simulink model "FOC_AM263X"  (R2024b)
settings: Solver=FixedStepAuto  StartTime=0.0  StopTime=10.0  RelTol=1e-3
model workspace: external: MATLAB File C:\Users\A0499511\Documents\MATLAB\Examples\R2024b\c2b\SensorlessfocUsingC2000ProcessorsExample\FOC_AM263X_Data.m (data not in the file)
values from neighbouring files (symbols this model uses):
  acceleration = 20000/PU_System.N_base    [FOC_AM263PX_Datascript.m]    (also in FOC_AM263X_Datascript.m)
  inverter = mcb_SetInverterParameters('BoostXL-DRV8305')    [FOC_AM263PX_Datascript.m]    (also in FOC_AM263X_Datascript.m)
  PI_params = mcb.internal.SetControllerParameters(pmsm,inverter,PU_System,T_pwm,2*Ts,Ts_speed)    [FOC_AM263PX_Datascript.m]    (also in FOC_AM263X_Datascript.m)
  pmsm = mcb_SetPMSMMotorParameters('BLY171D')    [FOC_AM263PX_Datascript.m]    (also in FOC_AM263X_Datascript.m)
  Speed_openLoop_PU = 0.1    [FOC_AM263PX_Datascript.m]    (also in FOC_AM263X_Datascript.m)
  T_Ref_openLoop = 1    [FOC_AM263PX_Datascript.m]    (also in FOC_AM263X_Datascript.m)
  target = mcb_SetProcessorDetails('F280049C',PWM_frequency)    [FOC_AM263PX_Datascript.m]
  Ts_motor = T_pwm/2    (= 2.5e-05)    [FOC_AM263PX_Datascript.m]    (also in FOC_AM263X_Datascript.m)
  Ts_simulink = T_pwm/2    (= 2.5e-05)    [FOC_AM263PX_Datascript.m]    (also in FOC_AM263X_Datascript.m)
  Ts_speed = 20*Ts    (= 0.001)    [FOC_AM263PX_Datascript.m]    (also in FOC_AM263X_Datascript.m)
undefined symbols (not defined in the file or in its folder): SYSCLOCKOUT
libraries: peripheral_library_blocks x13, simulink x5, HWI_lib x1, mcbplantlib x1, mcbcontrolslib x1, mcbpositiondecoderlib x1, autolibpmsmexterior x1
(part 3 of 3)

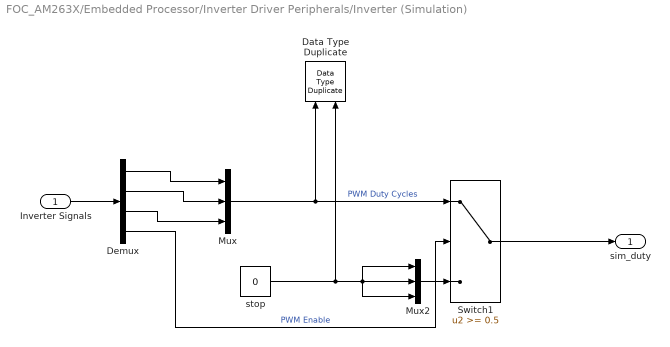
== system FOC_AM263X/Embedded Processor/Inverter Driver Peripherals/Inverter (Simulation) ==
  Inverter Signals : Inport
  Data Type Duplicate : DataTypeDuplicate
  Demux : Demux
  Mux : Mux  Inputs=3
  Mux2 : Mux  Inputs=3
  Switch1 : Switch  Threshold=0.5  RndMeth=Simplest  SaturateOnIntegerOverflow=off  InputSameDT=off
  stop : Constant  Value=0  OutDataTypeStr=Inherit: Inherit via back propagation
  sim_duty : Outport  VectorParamsAs1DForOutWhenUnconnected=off
  wires:
  stop/1 -> Data Type Duplicate/2, Mux2/1, Mux2/3, Mux2/2
  Mux2/1 -> Switch1/3
  Switch1/1 -> sim_duty/1
  Inverter Signals/1 -> Demux/1
  Demux/4 -> Switch1/2  "PWM Enable"
  Mux/1 -> Data Type Duplicate/1, Switch1/1  "PWM Duty Cycles"
  Demux/1 -> Mux/1
  Demux/2 -> Mux/2
  Demux/3 -> Mux/3

== system FOC_AM263X/Embedded Processor/Rate Limiter/Slew Rate ==
  In1 : Inport
  Speed_Ref : Inport  Port=2
  Merge : Merge
  Rate Limiter for FO : Subsystem  TreatAsAtomicUnit=on
  Rate Limiter for SMO : Subsystem  TreatAsAtomicUnit=on
  Switch Case : SwitchCase  CaseConditions={0,1}  ShowDefaultCase=off
  Out1 : Outport
  wires:
  Switch Case/1 -> Rate Limiter for SMO/Action
  Merge/1 -> Out1/1
  Rate Limiter for FO/1(Out1) -> Merge/2
  Speed_Ref/1 -> Rate Limiter for FO/1(Speed_Ref), Rate Limiter for SMO/1(Speed_Ref)
  Switch Case/2 -> Rate Limiter for FO/Action
  Rate Limiter for SMO/1(Out1) -> Merge/1
  In1/1 -> Switch Case/1

== system FOC_AM263X/Embedded Processor/SCI Interrupt/Code Generation ==
  Hardware Interrupt : HWI_lib/Hardware Interrupt  INTERRUPT_TYPE=UART  ISR_NUMBER=38  INSTANCE_NUMBER=0  SHOW_INPUTPORT=off
      settings: SourceProductName=Embedded Coder Support Package for AM263x - HWI Block
  HW_INT : Outport  VectorParamsAs1DForOutWhenUnconnected=off
  wires:
  Hardware Interrupt/1 -> HW_INT/1

== system FOC_AM263X/Embedded Processor/SCI Interrupt/Simulation ==
  SCI_Rx_INT : simulink/Ports & Subsystems/Function-Call Generator  sample_time=0.1  numberOfIterations=1  DisallowWideOutput=off
  HW_INT : Outport
  wires:
  SCI_Rx_INT/1 -> HW_INT/1

== system FOC_AM263X/Embedded Processor/Sensor Driver Blocks/Sensor Driver Blocks (codegen) ==
  Sim : Inport
  ADC : peripheral_library_blocks/ADC  ADCModule=ADC4  Prescaler=4.0  ResolutionMode=Twelve bit conversion  SOCPriority=All Round Robin  SignalMode=Sample on single pin with VREFLO  SOCTriggerNo=SOC0  SOCx_acquisition_Window=20  SOCxTriggerSource=EPWM2 SOCA  INTWillTriggerSOCx=No ADCINT Trigger  DataType=Unsigned INT16  ADCEnableConverter=on  PulseMode=Pulse generation at End of Acquisition Window  PostInterruptAtEOCTrigger=off  InterruptSelection=ADC Interrupt Number 1  InterruptSOCSource=SOC0  ADCINT1CONTINOUSMODE=off  ADCINT2CONTINOUSMODE=off  ADCINT3CONTINOUSMODE=off  ADCINT4CONTINOUSMODE=off  SampleTime=-1  Channels=Channel 4  Channels1=Channels 0 and 1  PPBBlock=PPB Block 1  PPBSocEocNO=SOC0  Enable_Event_ADC_Trip_High=off  Enable_Event_ADC_Trip_Low=off  Enable_Event_ADC_Zero_Crossing=off  Enable_Interrupt_Event_ADC_Trip_High=off  Enable_Interrupt_Event_ADC_Trip_Low=off  Enable_Interrupt_Event_ADC_Zero_Crossing=off  PPBEnableTwoComplement=off  PPBEnablePPBEventCBCClear=off  PPB_Calibration_Offset=0  PPB_Reference_Offset=0  PPB_High_Trip_Limit=0  PPB_Low_Trip_Limit=0  BurstModeTrigger=Software Source  BurstSize=1 SOC long  ADCEnableBurstMode=off
  ADC1 : peripheral_library_blocks/ADC  ADCModule=ADC0  Prescaler=4.0  ResolutionMode=Twelve bit conversion  SOCPriority=All Round Robin  SignalMode=Sample on single pin with VREFLO  SOCTriggerNo=SOC1  SOCx_acquisition_Window=20  SOCxTriggerSource=EPWM2 SOCA  INTWillTriggerSOCx=No ADCINT Trigger  DataType=Unsigned INT16  ADCEnableConverter=on  PulseMode=Pulse generation at End of Acquisition Window  PostInterruptAtEOCTrigger=off  InterruptSelection=ADC Interrupt Number 1  InterruptSOCSource=SOC1  ADCINT1CONTINOUSMODE=on  ADCINT2CONTINOUSMODE=off  ADCINT3CONTINOUSMODE=off  ADCINT4CONTINOUSMODE=off  SampleTime=-1  Channels=Channel 1  Channels1=Channels 0 and 1  PPBBlock=PPB Block 1  PPBSocEocNO=SOC0  Enable_Event_ADC_Trip_High=off  Enable_Event_ADC_Trip_Low=off  Enable_Event_ADC_Zero_Crossing=off  Enable_Interrupt_Event_ADC_Trip_High=off  Enable_Interrupt_Event_ADC_Trip_Low=off  Enable_Interrupt_Event_ADC_Zero_Crossing=off  PPBEnableTwoComplement=off  PPBEnablePPBEventCBCClear=off  PPB_Calibration_Offset=0  PPB_Reference_Offset=0  PPB_High_Trip_Limit=0  PPB_Low_Trip_Limit=0  BurstModeTrigger=Software Source  BurstSize=1 SOC long  ADCEnableBurstMode=off
  Mux1 : Mux  Inputs=2
  Terminator : Terminator
  out : Outport
  wires:
  Mux1/1 -> out/1
  Sim/1 -> Terminator/1
  ADC/1 -> Mux1/1
  ADC1/1 -> Mux1/2

== system FOC_AM263X/Embedded Processor/Sensor Driver Blocks/Sensor Driver Blocks (sim) ==
  Sim : Inport
  out : Outport
  wires:
  Sim/1 -> out/1

== system FOC_AM263X/Embedded Processor/Serial Receive/Code Generation ==
  MATLAB System : MATLABSystem  System=UART_READ  UARTPort=UART0  OutputDataLength=2  DataType=Unsigned int16  SampleTime=-1
      mask Type: UART_READ
      mask Display:
      | disp('UART_READ');
      | port_label('output',1,'UARTData');
  Data : Outport
  wires:
  MATLAB System/1 -> Data/1

== system FOC_AM263X/Embedded Processor/Serial Receive/Data_Conditioning ==
  In1 : Inport
  Data Type Conversion1 : DataTypeConversion  OutDataTypeStr=single  RndMeth=Simplest  SaturateOnIntegerOverflow=off
  Data Type Conversion2 : DataTypeConversion  OutDataTypeStr=fixdt(1,16,12)  ConvertRealWorld=Stored Integer (SI)  RndMeth=Simplest  SaturateOnIntegerOverflow=off
  Demux : Demux  Outputs=2
  Out1 : Outport  VectorParamsAs1DForOutWhenUnconnected=off
  Data : Outport  Port=2  VectorParamsAs1DForOutWhenUnconnected=off
  wires:
  Data Type Conversion1/1 -> Out1/1
  Data Type Conversion2/1 -> Data Type Conversion1/1
  In1/1 -> Demux/1
  Demux/1 -> Data Type Conversion2/1
  Demux/2 -> Data/1

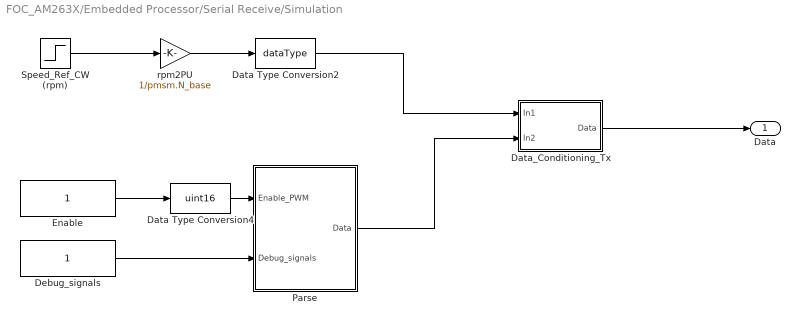
== system FOC_AM263X/Embedded Processor/Serial Receive/Simulation ==
  Data Type Conversion2 : DataTypeConversion  OutDataTypeStr=dataType  RndMeth=Simplest  SaturateOnIntegerOverflow=off
  Data Type Conversion4 : DataTypeConversion  OutDataTypeStr=uint16  RndMeth=Simplest  SaturateOnIntegerOverflow=off
  Data_Conditioning_Tx : Subsystem  VariantControl=~isequal(dataType, 'single')
  Debug_signals : Constant  OutDataTypeStr=uint16  SampleTime=-1
  Enable : Constant  OutDataTypeStr=dataType  SampleTime=-1
  Parse : Subsystem
  Speed_Ref_CW (rpm) : Step  Time=T_Ref_openLoop  Before=Speed_openLoop_PU*pmsm.N_base  After=0.5*pmsm.N_base
  rpm2PU : Gain  Gain=1/pmsm.N_base  RndMeth=Simplest  OutDataTypeStr=Inherit: Same as input
  Data : Outport
  wires:
  Data_Conditioning_Tx/1(Data) -> Data/1
  rpm2PU/1 -> Data Type Conversion2/1
  Enable/1 -> Data Type Conversion4/1
  Speed_Ref_CW (rpm)/1 -> rpm2PU/1
  Data Type Conversion4/1 -> Parse/1(Enable_PWM)
  Debug_signals/1 -> Parse/2(Debug_signals)
  Data Type Conversion2/1 -> Data_Conditioning_Tx/1(In1)
  Parse/1(Data) -> Data_Conditioning_Tx/2(In2)

== system FOC_AM263X/Embedded Processor/Serial Receive/unParse ==
  Data : Inport
  Bitwise Operator : simulink/Logic and Bit Operations/Bitwise Operator  logicop=AND  UseBitMask=on  BitMask=hex2dec('0001')  BitMaskRealWorld=Stored Integer
  Bitwise Operator1 : simulink/Logic and Bit Operations/Bitwise Operator  logicop=AND  UseBitMask=on  BitMask=hex2dec('00F0')  BitMaskRealWorld=Stored Integer
  Data Type Conversion3 : DataTypeConversion  OutDataTypeStr=boolean  RndMeth=Simplest  SaturateOnIntegerOverflow=off
  Data Type Conversion4 : DataTypeConversion  OutDataTypeStr=uint16  RndMeth=Simplest  SaturateOnIntegerOverflow=off
  Shift Arithmetic1 : ArithShift  BitShiftNumber=4
  Enable_PWM : Outport
  Debug_signals : Outport  Port=2
  wires:
  Bitwise Operator1/1 -> Shift Arithmetic1/1
  Data/1 -> Bitwise Operator/1, Bitwise Operator1/1
  Bitwise Operator/1 -> Data Type Conversion3/1
  Data Type Conversion4/1 -> Debug_signals/1
  Shift Arithmetic1/1 -> Data Type Conversion4/1
  Data Type Conversion3/1 -> Enable_PWM/1

== system FOC_AM263X/Inverter and Motor - Plant Model/Inverter and Motor - Plant Model/Codegeneration ==
  Duty_Cycles : Inport
  Ground : Ground
  Terminator : Terminator
  Feedbacks : Outport  VectorParamsAs1DForOutWhenUnconnected=off
  wires:
  Duty_Cycles/1 -> Terminator/1
  Ground/1 -> Feedbacks/1

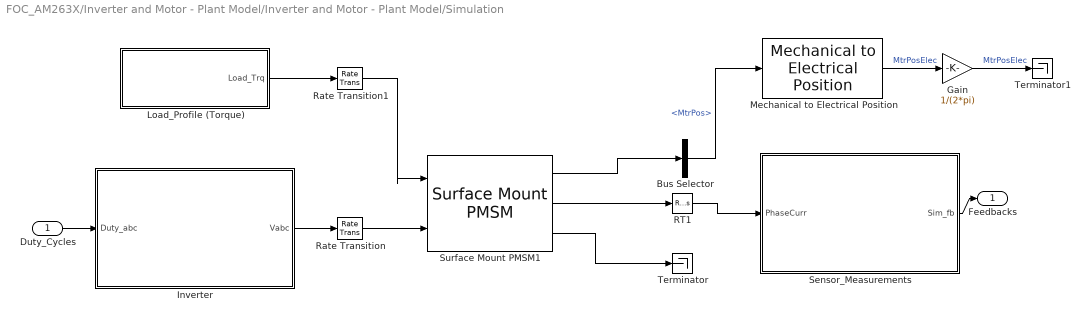
== system FOC_AM263X/Inverter and Motor - Plant Model/Inverter and Motor - Plant Model/Simulation ==
  Duty_Cycles : Inport
  Bus Selector : BusSelector  OutputSignals=MtrPos
  Gain : Gain  Gain=1/(2*pi)  OutDataTypeStr=Inherit: Same as input
  Inverter : Subsystem
  Load_Profile (Torque) : Subsystem
  Mechanical to Electrical Position : mcbpositiondecoderlib/Mechanical to Electrical Position  PolePairsInputType=Specify via dialog  NrPP=pmsm.p  selectedRange=Radians  MechOfstInputType=Specify via dialog  mechOffsetIn=0  maxAngleIn=2*pi  InputDataType=single  VariantSelect=floating-point
  RT1 : RateTransition  Deterministic=off  OutPortSampleTime=Ts_simulink
  Rate Transition : RateTransition  Deterministic=off  OutPortSampleTime=Ts_motor
  Rate Transition1 : RateTransition  Deterministic=off  OutPortSampleTime=Ts_motor
  Sensor_Measurements : Subsystem
  Surface Mount PMSM1 : autolibpmsmexterior/Surface Mount PMSM  port_config=Torque  sim_type=Discrete  Ts=Ts_motor  P=pmsm.p  Rs=pmsm.Rs + inverter.R_board  Ldq_=pmsm.Ld  KConstText=Permanent flux linkage constant (lambda_pm):  lambda_pm=pmsm.FluxPM  Ke=159.9771  Kt=1.323  mechanical=[pmsm.J, pmsm.B, 0]  idq0=[0 0]  theta_init=0  omega_init=0  KConst=pmsm.FluxPM  lambda_pm_calc=pmsm.FluxPM  RefBlkName='autolibpmsmexterior/Surface Mount PMSM'  aMode=5  Ldq="[0.0017      0.0017]"
  Terminator : Terminator
  Terminator1 : Terminator
  Feedbacks : Outport  VectorParamsAs1DForOutWhenUnconnected=off
  wires:
  RT1/1 -> Sensor_Measurements/1(PhaseCurr)
  Load_Profile (Torque)/1(Load_Trq) -> Rate Transition1/1
  Sensor_Measurements/1(Sim_fb) -> Feedbacks/1
  Gain/1 -> Terminator1/1  "MtrPosElec"
  Inverter/1(Vabc) -> Rate Transition/1
  Mechanical to Electrical Position/1 -> Gain/1  "MtrPosElec"
  Duty_Cycles/1 -> Inverter/1(Duty_abc)
  Bus Selector/1 -> Mechanical to Electrical Position/1  "<MtrPos>"
  Rate Transition1/1 -> Surface Mount PMSM1/1
  Rate Transition/1 -> Surface Mount PMSM1/2
  Surface Mount PMSM1/1 -> Bus Selector/1
  Surface Mount PMSM1/2 -> RT1/1
  Surface Mount PMSM1/3 -> Terminator/1

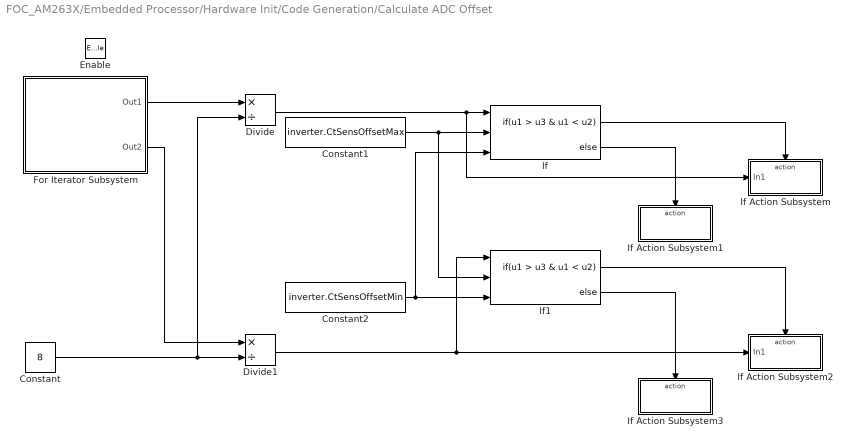
== system FOC_AM263X/Embedded Processor/Hardware Init/Code Generation/Calculate ADC Offset  ==
  Enable : EnablePort
  Constant : Constant  Value=8
  Constant1 : Constant  Value=inverter.CtSensOffsetMax  OutDataTypeStr=Inherit: Inherit via back propagation
  Constant2 : Constant  Value=inverter.CtSensOffsetMin  OutDataTypeStr=Inherit: Inherit via back propagation
  Divide : Product  Inputs=*/  OutDataTypeStr=uint16
  Divide1 : Product  Inputs=*/  OutDataTypeStr=uint16
  For Iterator Subsystem : Subsystem  TreatAsAtomicUnit=on
  If : If  NumInputs=3  IfExpression=u1 > u3 & u1 < u2
  If Action Subsystem : Subsystem  TreatAsAtomicUnit=on
  If Action Subsystem1 : Subsystem  TreatAsAtomicUnit=on
  If Action Subsystem2 : Subsystem  TreatAsAtomicUnit=on
  If Action Subsystem3 : Subsystem  TreatAsAtomicUnit=on
  If1 : If  NumInputs=3  IfExpression=u1 > u3 & u1 < u2
  wires:
  For Iterator Subsystem/1(Out1) -> Divide/1
  If1/2 -> If Action Subsystem3/Action
  If1/1 -> If Action Subsystem2/Action
  If/2 -> If Action Subsystem1/Action
  For Iterator Subsystem/2(Out2) -> Divide1/1
  If/1 -> If Action Subsystem/Action
  Constant2/1 -> If/3, If1/3
  Constant1/1 -> If/2, If1/2
  Divide1/1 -> If1/1, If Action Subsystem2/1(In1)
  Constant/1 -> Divide/2, Divide1/2
  Divide/1 -> If Action Subsystem/1(In1), If/1

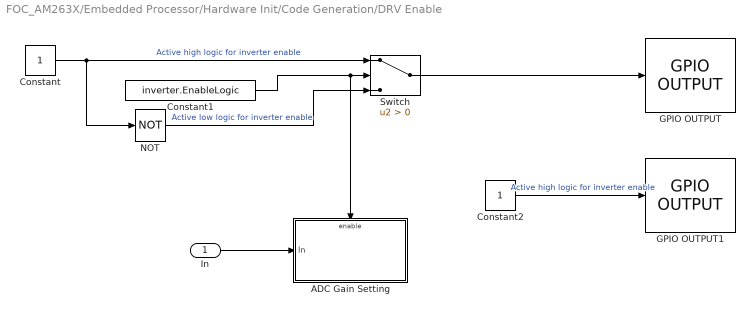
== system FOC_AM263X/Embedded Processor/Hardware Init/Code Generation/DRV Enable ==
  In : Inport
  ADC Gain Setting : Subsystem
  Constant : Constant  OutDataTypeStr=Inherit: Inherit via back propagation
  Constant1 : Constant  Value=inverter.EnableLogic
  Constant2 : Constant  OutDataTypeStr=Inherit: Inherit via back propagation
  GPIO OUTPUT : peripheral_library_blocks/GPIO OUTPUT  GPIO_Pin=GPIO87  Trigger_Type=None  GPIOEnableInterrupt=off
  GPIO OUTPUT1 : peripheral_library_blocks/GPIO OUTPUT  GPIO_Pin=GPIO64  Trigger_Type=None  GPIOEnableInterrupt=off
  NOT : Logic  Operator=NOT  IconShape=distinctive  AllPortsSameDT=off  OutDataTypeStr=boolean
  Switch : Switch  Criteria=u2 > Threshold  SaturateOnIntegerOverflow=off  InputSameDT=off
  wires:
  NOT/1 -> Switch/3  "Active low logic for inverter enable"
  Constant/1 -> Switch/1, NOT/1  "Active high logic for inverter enable"
  Constant1/1 -> ADC Gain Setting/Enable, Switch/2
  Switch/1 -> GPIO OUTPUT/1
  Constant2/1 -> GPIO OUTPUT1/1  "Active high logic for inverter enable"
  In/1 -> ADC Gain Setting/1(In)

== system FOC_AM263X/Embedded Processor/Hardware Init/Code Generation/Default ADC Offset ==
  Enable : EnablePort
  Constant : Constant  Value=inverter.CtSensAOffset  OutDataTypeStr=Inherit: Inherit via back propagation
  Constant1 : Constant  Value=inverter.CtSensBOffset  OutDataTypeStr=Inherit: Inherit via back propagation
  Data Store Write1 : DataStoreWrite  DataStoreName=IaOffset  IndexOptions=Index vector (dialog)  Indices=1  OutputSizes=1
  Data Store Write2 : DataStoreWrite  DataStoreName=IbOffset  IndexOptions=Index vector (dialog)  Indices=1  OutputSizes=1
  wires:
  Constant/1 -> Data Store Write1/1
  Constant1/1 -> Data Store Write2/1

== system FOC_AM263X/Embedded Processor/Rate Limiter/Slew Rate/Rate Limiter for FO ==
  Speed_Ref : Inport
  Action Port : ActionPort  ActionPortLabel=case [ 1 ]:
  Out1 : Outport
  wires:
  Speed_Ref/1 -> Out1/1

== system FOC_AM263X/Embedded Processor/Rate Limiter/Slew Rate/Rate Limiter for SMO ==
  Speed_Ref : Inport
  Action Port : ActionPort  ActionPortLabel=case [ 0 ]:
  Rate Limiter : RateLimiter  RisingSlewLimit=acceleration  FallingSlewLimit=-acceleration  SampleTimeMode=inherited  InitialCondition=Speed_openLoop_PU
  Rate Limiter1 : RateLimiter  RisingSlewLimit=acceleration  FallingSlewLimit=-acceleration  SampleTimeMode=inherited  InitialCondition=-Speed_openLoop_PU
  Switch : Switch  SaturateOnIntegerOverflow=off  InputSameDT=off
  Out1 : Outport
  wires:
  Speed_Ref/1 -> Rate Limiter/1, Rate Limiter1/1, Switch/2
  Switch/1 -> Out1/1
  Rate Limiter1/1 -> Switch/3
  Rate Limiter/1 -> Switch/1

== system FOC_AM263X/Embedded Processor/Serial Receive/Simulation/Data_Conditioning_Tx ==
  In1 : Inport
  In2 : Inport  Port=2
  Data Type Conversion : DataTypeConversion  OutDataTypeStr=fixdt(1,16,12)  RndMeth=Simplest  SaturateOnIntegerOverflow=off
  Data Type Conversion3 : DataTypeConversion  OutDataTypeStr=uint16  ConvertRealWorld=Stored Integer (SI)  RndMeth=Simplest  SaturateOnIntegerOverflow=off
  Mux : Mux  Inputs=2
  Data : Outport
  wires:
  In1/1 -> Data Type Conversion/1
  Data Type Conversion3/1 -> Mux/1
  Data Type Conversion/1 -> Data Type Conversion3/1
  In2/1 -> Mux/2
  Mux/1 -> Data/1

== system FOC_AM263X/Embedded Processor/Serial Receive/Simulation/Parse ==
  Enable_PWM : Inport
  Debug_signals : Inport  Port=2
  Bitwise Operator : simulink/Logic and Bit Operations/Bitwise Operator  logicop=AND  UseBitMask=on  BitMask=hex2dec('0001')  BitMaskRealWorld=Stored Integer
  Bitwise Operator1 : simulink/Logic and Bit Operations/Bitwise Operator  logicop=AND  UseBitMask=on  BitMask=hex2dec('00F0')  BitMaskRealWorld=Stored Integer
  Shift Arithmetic1 : ArithShift  BitShiftNumber=-4
  Sum : Sum  Inputs=|++
  Data : Outport
  wires:
  Bitwise Operator/1 -> Sum/1
  Debug_signals/1 -> Shift Arithmetic1/1
  Sum/1 -> Data/1
  Shift Arithmetic1/1 -> Bitwise Operator1/1
  Enable_PWM/1 -> Bitwise Operator/1
  Bitwise Operator1/1 -> Sum/2

== system FOC_AM263X/Inverter and Motor - Plant Model/Inverter and Motor - Plant Model/Simulation/Inverter ==
  Duty_abc : Inport
  Average-Value Inverter : mcbplantlib/Average-Value Inverter
  Constant2 : Constant  Value=inverter.V_dc  OutDataTypeStr=single  SampleTime=-1
  Data Type Conversion1 : DataTypeConversion  OutDataTypeStr=single  RndMeth=Simplest  SaturateOnIntegerOverflow=off
  Rate Transition3 : RateTransition  Deterministic=off  OutPortSampleTime=Ts_inverter
  Vabc : Outport  VectorParamsAs1DForOutWhenUnconnected=off
  wires:
  Constant2/1 -> Average-Value Inverter/2
  Data Type Conversion1/1 -> Rate Transition3/1
  Duty_abc/1 -> Data Type Conversion1/1
  Average-Value Inverter/1 -> Vabc/1
  Rate Transition3/1 -> Average-Value Inverter/1

== system FOC_AM263X/Inverter and Motor - Plant Model/Inverter and Motor - Plant Model/Simulation/Load_Profile (Torque) ==
  Data Type Conversion : DataTypeConversion  OutDataTypeStr=single  SaturateOnIntegerOverflow=off  RndMeth=Floor
  IIR Filter : mcbcontrolslib/IIR Filter  VariantControl=Low Pass Filter  VariantSelect=Low-pass  FilterConstantInputType=Specify via dialog  Filter_constant=0.0001  advancedSettings=off  Ts=50e-6  cutOff_freq=0.31834
  T_load : Step  Time=4  Before=0.05*pmsm.T_rated  After=0.5*pmsm.T_rated  SampleTime=Ts_simulink
  Load_Trq : Outport  VectorParamsAs1DForOutWhenUnconnected=off
  wires:
  Data Type Conversion/1 -> IIR Filter/1
  IIR Filter/1 -> Load_Trq/1
  T_load/1 -> Data Type Conversion/1

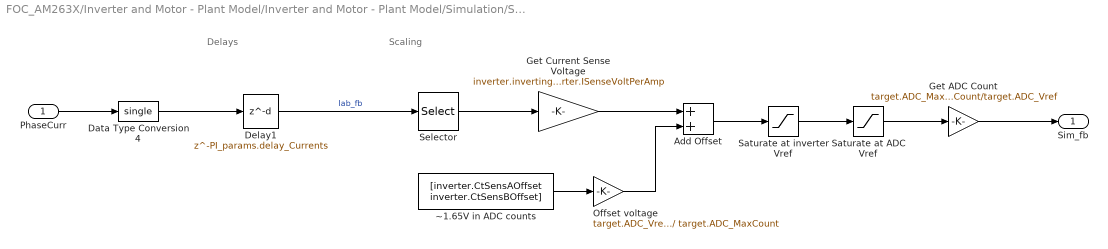
== system FOC_AM263X/Inverter and Motor - Plant Model/Inverter and Motor - Plant Model/Simulation/Sensor_Measurements ==
  note: Scaling
  note: Delays
  PhaseCurr : Inport
  Add Offset : Sum  RndMeth=Simplest
  Data Type Conversion4 : DataTypeConversion  OutDataTypeStr=single  RndMeth=Simplest  SaturateOnIntegerOverflow=off
  Delay1 : Delay  DelayLength=PI_params.delay_Currents
  Get ADC Count : Gain  Gain=target.ADC_MaxCount/target.ADC_Vref  OutMin=0  OutMax=target.ADC_MaxCount  OutDataTypeStr=uint16  RndMeth=Simplest
  Get Current Sense Voltage : Gain  Gain=inverter.invertingAmp * inverter.ISenseVoltPerAmp  RndMeth=Simplest  OutDataTypeStr=Inherit: Same as input
  Offset voltage : Gain  Gain=target.ADC_Vref / target.ADC_MaxCount  RndMeth=Simplest
  Saturate at ADC Vref : Saturate  UpperLimit=target.ADC_Vref  LowerLimit=0
  Saturate at inverter Vref : Saturate  UpperLimit=inverter.ISenseVref  LowerLimit=0
  Selector : Selector  InputPortWidth=3  IndexOptions=Index vector (dialog)  Indices=[1 2]  OutputSizes=1
  ~1.65V in ADC counts : Constant  Value=[inverter.CtSensAOffset inverter.CtSensBOffset]  OutDataTypeStr=uint16  SampleTime=-1
  Sim_fb : Outport  VectorParamsAs1DForOutWhenUnconnected=off
  wires:
  Delay1/1 -> Selector/1  "Iab_fb"
  Data Type Conversion4/1 -> Delay1/1
  PhaseCurr/1 -> Data Type Conversion4/1
  Add Offset/1 -> Saturate at inverter Vref/1
  Saturate at inverter Vref/1 -> Saturate at ADC Vref/1
  ~1.65V in ADC counts/1 -> Offset voltage/1
  Get Current Sense Voltage/1 -> Add Offset/1
  Saturate at ADC Vref/1 -> Get ADC Count/1
  Selector/1 -> Get Current Sense Voltage/1
  Offset voltage/1 -> Add Offset/2
  Get ADC Count/1 -> Sim_fb/1

== system FOC_AM263X/Embedded Processor/Hardware Init/Code Generation/Calculate ADC Offset /For Iterator Subsystem ==
  ADC : peripheral_library_blocks/ADC  ADCModule=ADC4  Prescaler=2.0  ResolutionMode=Twelve bit conversion  SOCPriority=All Round Robin  SignalMode=Sample on single pin with VREFLO  SOCTriggerNo=SOC2  SOCx_acquisition_Window=16  SOCxTriggerSource=Software Source  INTWillTriggerSOCx=No ADCINT Trigger  DataType=Unsigned INT16  ADCEnableConverter=on  PulseMode=Pulse generation at End of Acquisition Window  PostInterruptAtEOCTrigger=off  InterruptSelection=ADC Interrupt Number 1  InterruptSOCSource=SOC0  ADCINT1CONTINOUSMODE=off  ADCINT2CONTINOUSMODE=off  ADCINT3CONTINOUSMODE=off  ADCINT4CONTINOUSMODE=off  SampleTime=-1  Channels=Channel 4  Channels1=Channels 0 and 1  PPBBlock=PPB Block 1  PPBSocEocNO=SOC0  Enable_Event_ADC_Trip_High=off  Enable_Event_ADC_Trip_Low=off  Enable_Event_ADC_Zero_Crossing=off  Enable_Interrupt_Event_ADC_Trip_High=off  Enable_Interrupt_Event_ADC_Trip_Low=off  Enable_Interrupt_Event_ADC_Zero_Crossing=off  PPBEnableTwoComplement=off  PPBEnablePPBEventCBCClear=off  PPB_Calibration_Offset=0  PPB_Reference_Offset=0  PPB_High_Trip_Limit=0  PPB_Low_Trip_Limit=0  BurstModeTrigger=Software Source  BurstSize=1 SOC long  ADCEnableBurstMode=off
  ADC1 : peripheral_library_blocks/ADC  ADCModule=ADC0  Prescaler=2.0  ResolutionMode=Twelve bit conversion  SOCPriority=All Round Robin  SignalMode=Sample on single pin with VREFLO  SOCTriggerNo=SOC3  SOCx_acquisition_Window=16  SOCxTriggerSource=Software Source  INTWillTriggerSOCx=No ADCINT Trigger  DataType=Unsigned INT16  ADCEnableConverter=on  PulseMode=Pulse generation at End of Acquisition Window  PostInterruptAtEOCTrigger=off  InterruptSelection=ADC Interrupt Number 1  InterruptSOCSource=SOC0  ADCINT1CONTINOUSMODE=off  ADCINT2CONTINOUSMODE=off  ADCINT3CONTINOUSMODE=off  ADCINT4CONTINOUSMODE=off  SampleTime=-1  Channels=Channel 1  Channels1=Channels 0 and 1  PPBBlock=PPB Block 1  PPBSocEocNO=SOC0  Enable_Event_ADC_Trip_High=off  Enable_Event_ADC_Trip_Low=off  Enable_Event_ADC_Zero_Crossing=off  Enable_Interrupt_Event_ADC_Trip_High=off  Enable_Interrupt_Event_ADC_Trip_Low=off  Enable_Interrupt_Event_ADC_Zero_Crossing=off  PPBEnableTwoComplement=off  PPBEnablePPBEventCBCClear=off  PPB_Calibration_Offset=0  PPB_Reference_Offset=0  PPB_High_Trip_Limit=0  PPB_Low_Trip_Limit=0  BurstModeTrigger=Software Source  BurstSize=1 SOC long  ADCEnableBurstMode=off
  For Iterator : ForIterator  IterationLimit=16  IterationVariableDataType=uint16
  If : If  IfExpression=u1 > 8  ShowElse=off
  If Action Subsystem : Subsystem  TreatAsAtomicUnit=on
  Out1 : Outport
  Out2 : Outport  Port=2
  wires:
  For Iterator/1 -> If/1
  If Action Subsystem/1(Out1) -> Out1/1
  If Action Subsystem/2(Out2) -> Out2/1
  If/1 -> If Action Subsystem/Action
  ADC/1 -> If Action Subsystem/1(In1)
  ADC1/1 -> If Action Subsystem/2(In2)

== system FOC_AM263X/Embedded Processor/Hardware Init/Code Generation/Calculate ADC Offset /If Action Subsystem ==
  In1 : Inport
  Action Port : ActionPort  ActionPortLabel=if(u1 > u3 & u1 < u2)
  Data Store Write1 : DataStoreWrite  DataStoreName=IaOffset  IndexOptions=Index vector (dialog)  Indices=1  OutputSizes=1
  wires:
  In1/1 -> Data Store Write1/1

== system FOC_AM263X/Embedded Processor/Hardware Init/Code Generation/Calculate ADC Offset /If Action Subsystem1 ==
  Action Port : ActionPort  ActionPortLabel=else
  Constant : Constant  Value=inverter.CtSensAOffset  OutDataTypeStr=Inherit: Inherit via back propagation
  Data Store Write1 : DataStoreWrite  DataStoreName=IaOffset  IndexOptions=Index vector (dialog)  Indices=1  OutputSizes=1
  wires:
  Constant/1 -> Data Store Write1/1

== system FOC_AM263X/Embedded Processor/Hardware Init/Code Generation/Calculate ADC Offset /If Action Subsystem2 ==
  In1 : Inport
  Action Port : ActionPort  ActionPortLabel=if(u1 > u3 & u1 < u2)
  Data Store Write2 : DataStoreWrite  DataStoreName=IbOffset  IndexOptions=Index vector (dialog)  Indices=1  OutputSizes=1
  wires:
  In1/1 -> Data Store Write2/1

== system FOC_AM263X/Embedded Processor/Hardware Init/Code Generation/Calculate ADC Offset /If Action Subsystem3 ==
  Action Port : ActionPort  ActionPortLabel=else
  Constant1 : Constant  Value=inverter.CtSensBOffset  OutDataTypeStr=Inherit: Inherit via back propagation
  Data Store Write2 : DataStoreWrite  DataStoreName=IbOffset  IndexOptions=Index vector (dialog)  Indices=1  OutputSizes=1
  wires:
  Constant1/1 -> Data Store Write2/1

== system FOC_AM263X/Embedded Processor/Hardware Init/Code Generation/DRV Enable/ADC Gain Setting ==
  In : Inport
  Enable : EnablePort
  Demux : Demux  Outputs=2
  Display : Display
      settings: Format=hex (Stored Integer)
  Display1 : Display
      settings: Format=hex (Stored Integer)
  MCSPI CONTROLLER TRANSFER : peripheral_library_blocks/MCSPI CONTROLLER TRANSFER  MCSPI_Instance=MCSPI1  Enable_Channel0=on  Enable_Channel1=off  Output_Data_Length=1  Channel0_Data_Size=16  Channel0_Auto_CSDeassert=on  Channel1_Data_Size=8  Channel1_Auto_CSDeassert=on
  MCSPI CONTROLLER TRANSFER1 : peripheral_library_blocks/MCSPI CONTROLLER TRANSFER  MCSPI_Instance=MCSPI1  Enable_Channel0=on  Enable_Channel1=off  Output_Data_Length=1  Channel0_Data_Size=16  Channel0_Auto_CSDeassert=on  Channel1_Data_Size=8  Channel1_Auto_CSDeassert=on
  wires:
  In/1 -> Demux/1
  Demux/1 -> MCSPI CONTROLLER TRANSFER/1
  MCSPI CONTROLLER TRANSFER/1 -> Display/1
  Demux/2 -> MCSPI CONTROLLER TRANSFER1/1
  MCSPI CONTROLLER TRANSFER1/1 -> Display1/1

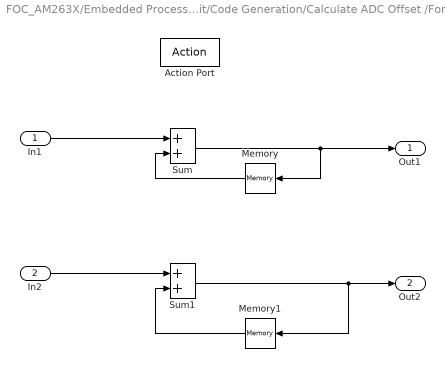
== system FOC_AM263X/Embedded Processor/Hardware Init/Code Generation/Calculate ADC Offset /For Iterator Subsystem/If Action Subsystem ==
  In1 : Inport
  In2 : Inport  Port=2
  Action Port : ActionPort  ActionPortLabel=if(u1 > 8)
  Memory : Memory  InheritSampleTime=on
  Memory1 : Memory  InheritSampleTime=on
  Sum : Sum
  Sum1 : Sum
  Out1 : Outport
  Out2 : Outport  Port=2
  wires:
  In1/1 -> Sum/1
  Sum/1 -> Out1/1, Memory/1
  In2/1 -> Sum1/1
  Memory/1 -> Sum/2
  Sum1/1 -> Out2/1, Memory1/1
  Memory1/1 -> Sum1/2
